simulink model "diagrama_LTI_desagragado"  (R2020b)
settings: Solver=VariableStepAuto  StartTime=0.0  StopTime=1.3  RelTol=1e-3
model workspace (MAT data in the model file):
  Cts = 0.818
  Jeq = 5.65099476805e-06
  Ld = 0.0066
  Lls = 0.0008
  Lq = 0.0058
  Pp = 3
  Rs = 1.02
  Rts_amb = 146.7
  beq = 1.5e-05
  lambda_m = 0.01546
  r = 314.3008
undefined symbols (not defined in the file or in its folder): sigbuilder_block
settings Model: Creator=Matias  LastModifiedBy=Matias

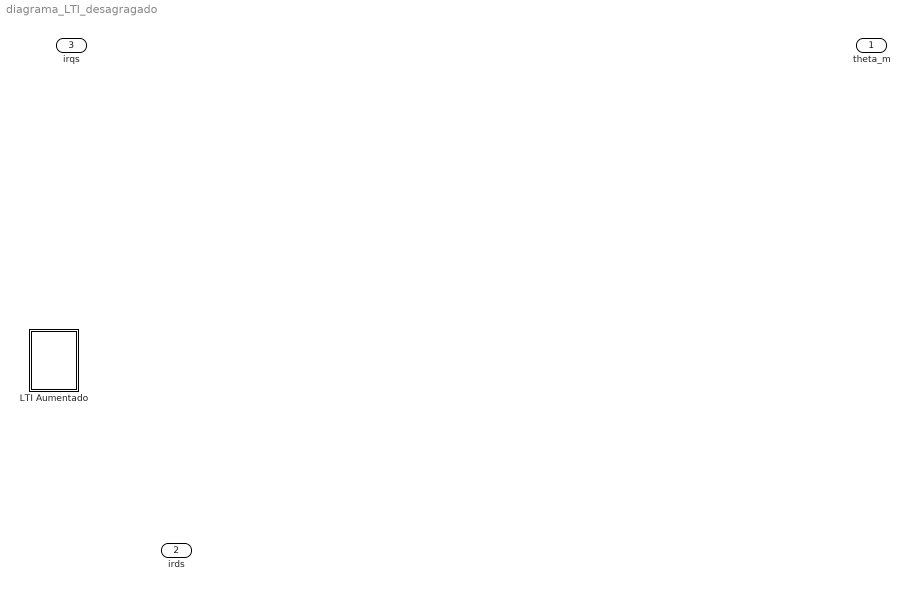
== system diagrama_LTI_desagragado ==
  LTI Aumentado : Subsystem
  theta_m : Outport
  irds : Outport  Port=2
  irqs : Outport  Port=3

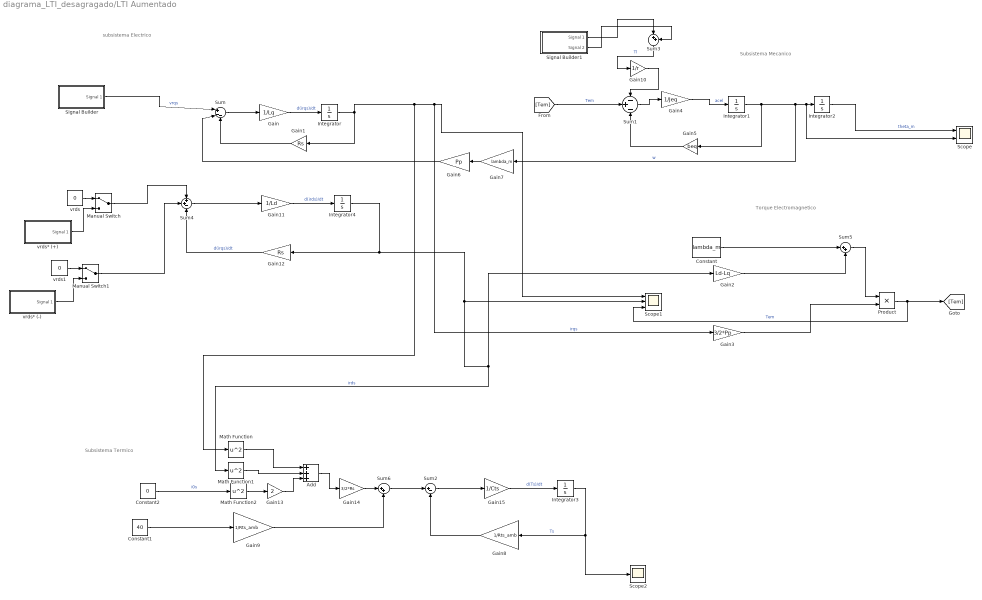
== system diagrama_LTI_desagragado/LTI Aumentado ==
  note: Subsistema Mecanico
  note: subsistema Electrico
  note: Subsistema Termico
  note: Torque Electromagnetico
  Add : Sum  Inputs=+++
  Constant : Constant  Value=lambda_m
  Constant1 : Constant  Value=40
  Constant2 : Constant  Value=0
  Gain : Gain  Gain=1/Lq
  Gain1 : Gain  Gain=Rs
  Gain10 : Gain  Gain=1/r
  Gain11 : Gain  Gain=1/Ld
  Gain12 : Gain  Gain=Rs
  Gain13 : Gain  Gain=2
  Gain14 : Gain  Gain=3/2*Rs
  Gain15 : Gain  Gain=1/Cts
  Gain2 : Gain  Gain=Ld-Lq
  Gain3 : Gain  Gain=3/2*Pp
  Gain4 : Gain  Gain=1/Jeq
  Gain5 : Gain  Gain=beq
  Gain6 : Gain  Gain=Pp
  Gain7 : Gain  Gain=lambda_m
  Gain8 : Gain  Gain=1/Rts_amb
  Gain9 : Gain  Gain=1/Rts_amb
  Integrator{,1..2,4} (4 alike) : Integrator
  Integrator3 : Integrator  InitialCondition=40
  Manual Switch : ManualSwitch
  Manual Switch1 : ManualSwitch
  Math Function : Math  Operator=square  SaturateOnIntegerOverflow=on
  Math Function1 : Math  Operator=square  SaturateOnIntegerOverflow=on
  Math Function2 : Math  Operator=square  SaturateOnIntegerOverflow=on
  Product : Product
  Scope : Scope  NumInputPorts=2
  Scope1 : Scope  NumInputPorts=3
  Scope2 : Scope
  Signal Builder : Subsystem  Tag=STV Subsys  LoadFcn=sigbuilder_block('load');  StartFcn=sigbuilder_block('start');  StopFcn=sigbuilder_block('stop');  ClipboardFcn=sigbuilder_block('clipboard');  mask(Sigbuilder block){tuvar=[0:10]}
      mask help: Simulink:masks:SigbuilderBlock_MD
      mask init:
      | if ~strcmp(get_param(bdroot(gcbh),'SimulationStatus'),'stopped') tuvar = sigbuilder_block('maskInit'); end
      settings: CopyFcn=sigbuilder_block('copy');  DeleteFcn=sigbuilder_block('delete');  ModelCloseFcn=sigbuilder_block('modelClose');  PreSaveFcn=sigbuilder_block('preSave');  PauseFcn=sigbuilder_block('pause');  ContinueFcn=sigbuilder_block('continue');  NameChangeFcn=sigbuilder_block('namechange');  OpenFcn=sigbuilder_block('open',[437.6 199.2 550.4 400 ]);  CloseFcn=sigbuilder_block('close');
      mask Display: plot(0, 0, 100, 100,[2, 2, 32, 32, 2], [68, 8, 8, 68, 68],[32, 2], [38, 38], [32, 19, 2],[53, 60, 44], [32, 17, 17, 2],[16, 16, 31, 31]);txt = getActiveGroup(gcbh);text(2, 100, txt,'verticalAlignment', 'top');
  Signal Builder1 : Subsystem  Tag=STV Subsys  LoadFcn=sigbuilder_block('load');  StartFcn=sigbuilder_block('start');  StopFcn=sigbuilder_block('stop');  ClipboardFcn=sigbuilder_block('clipboard');  mask(Sigbuilder block){tuvar=[0:10]}
      mask help: Simulink:masks:SigbuilderBlock_MD
      mask init:
      | if ~strcmp(get_param(bdroot(gcbh),'SimulationStatus'),'stopped') tuvar = sigbuilder_block('maskInit'); end
      settings: CopyFcn=sigbuilder_block('copy');  DeleteFcn=sigbuilder_block('delete');  ModelCloseFcn=sigbuilder_block('modelClose');  PreSaveFcn=sigbuilder_block('preSave');  PauseFcn=sigbuilder_block('pause');  ContinueFcn=sigbuilder_block('continue');  NameChangeFcn=sigbuilder_block('namechange');  OpenFcn=sigbuilder_block('open',[437.6 199.2 550.4 400 ]);  CloseFcn=sigbuilder_block('close');
      mask Display: plot(0, 0, 100, 100,[2, 2, 32, 32, 2], [68, 8, 8, 68, 68],[32, 2], [38, 38], [32, 19, 2],[53, 60, 44], [32, 17, 17, 2],[16, 16, 31, 31]);txt = getActiveGroup(gcbh);text(2, 100, txt,'verticalAlignment', 'top');
  Sum : Sum  Inputs=|+--
  Sum1 : Sum  Inputs=-+-
  Sum2 : Sum  Inputs=|+-
  Sum3 : Sum  Inputs=|++
  Sum4 : Sum  Inputs=++-
  Sum5 : Sum  Inputs=|++
  Sum6 : Sum  Inputs=|++
  vrds : Constant  Value=0
  vrds* (+) : Subsystem  Tag=STV Subsys  LoadFcn=sigbuilder_block('load');  StartFcn=sigbuilder_block('start');  StopFcn=sigbuilder_block('stop');  ClipboardFcn=sigbuilder_block('clipboard');  mask(Sigbuilder block){tuvar=[0:10]}
      mask help: Simulink:masks:SigbuilderBlock_MD
      mask init:
      | if ~strcmp(get_param(bdroot(gcbh),'SimulationStatus'),'stopped') tuvar = sigbuilder_block('maskInit'); end
      settings: CopyFcn=sigbuilder_block('copy');  DeleteFcn=sigbuilder_block('delete');  ModelCloseFcn=sigbuilder_block('modelClose');  PreSaveFcn=sigbuilder_block('preSave');  PauseFcn=sigbuilder_block('pause');  ContinueFcn=sigbuilder_block('continue');  NameChangeFcn=sigbuilder_block('namechange');  OpenFcn=sigbuilder_block('open',[437.6 199.2 550.4 400 ]);  CloseFcn=sigbuilder_block('close');
      mask Display: plot(0, 0, 100, 100,[2, 2, 32, 32, 2], [68, 8, 8, 68, 68],[32, 2], [38, 38], [32, 19, 2],[53, 60, 44], [32, 17, 17, 2],[16, 16, 31, 31]);txt = getActiveGroup(gcbh);text(2, 100, txt,'verticalAlignment', 'top');
  vrds* (-) : Subsystem  Tag=STV Subsys  LoadFcn=sigbuilder_block('load');  StartFcn=sigbuilder_block('start');  StopFcn=sigbuilder_block('stop');  ClipboardFcn=sigbuilder_block('clipboard');  mask(Sigbuilder block){tuvar=[0:10]}
      mask help: Simulink:masks:SigbuilderBlock_MD
      mask init:
      | if ~strcmp(get_param(bdroot(gcbh),'SimulationStatus'),'stopped') tuvar = sigbuilder_block('maskInit'); end
      settings: CopyFcn=sigbuilder_block('copy');  DeleteFcn=sigbuilder_block('delete');  ModelCloseFcn=sigbuilder_block('modelClose');  PreSaveFcn=sigbuilder_block('preSave');  PauseFcn=sigbuilder_block('pause');  ContinueFcn=sigbuilder_block('continue');  NameChangeFcn=sigbuilder_block('namechange');  OpenFcn=sigbuilder_block('open',[437.6 199.2 550.4 400 ]);  CloseFcn=sigbuilder_block('close');
      mask Display: plot(0, 0, 100, 100,[2, 2, 32, 32, 2], [68, 8, 8, 68, 68],[32, 2], [38, 38], [32, 19, 2],[53, 60, 44], [32, 17, 17, 2],[16, 16, 31, 31]);txt = getActiveGroup(gcbh);text(2, 100, txt,'verticalAlignment', 'top');
  vrds1 : Constant  Value=0
  wires:
  Gain7/1 -> Gain6/1
  Sum/1 -> Gain/1
  Integrator1/1 -> Gain7/1, Scope/2, Integrator2/1, Gain5/1  "w"
  Gain3/1 -> Product/2
  Integrator2/1 -> Scope/1  "theta_m"
  Gain15/1 -> Integrator3/1  "d(Ts)/dt"
  Integrator/1 -> Math Function/1, Gain3/1, Scope1/1, Gain1/1  "irqs"
  Gain4/1 -> Integrator1/1  "acel"
  Constant1/1 -> Gain9/1
  Gain5/1 -> Sum1/3
  Integrator4/1 -> Math Function1/1, Gain2/1, Scope1/2, Gain12/1  "irds"
  Sum4/1 -> Gain11/1
  Gain6/1 -> Sum/2
  Sum3/1 -> Gain10/1  "Tl"
  Gain11/1 -> Integrator4/1  "d(irds)/dt"
  Gain2/1 -> Sum5/2
  Constant/1 -> Sum5/1
  vrds* (+)/1(Signal 1) -> Manual Switch/2
  Sum2/1 -> Gain15/1
  vrds/1 -> Manual Switch/1
  Manual Switch/1 -> Sum4/1
  Gain14/1 -> Sum6/1
  Signal Builder1/1(Signal 1) -> Sum3/1
  Gain13/1 -> Add/3
  Product/1 -> Scope1/3, [Tem]  "Tem"
  vrds1/1 -> Manual Switch1/1
  Gain12/1 -> Sum4/3  "d(irqs)/dt"
  Gain10/1 -> Sum1/1
  Gain8/1 -> Sum2/2
  vrds* (-)/1(Signal 1) -> Manual Switch1/2
  Integrator3/1 -> Gain8/1, Scope2/1  "Ts"
  Signal Builder/1(Signal 1) -> Sum/1  "vrqs"
  Manual Switch1/1 -> Sum4/2
  Add/1 -> Gain14/1
  Signal Builder1/2(Signal 2) -> Sum3/2
  Math Function1/1 -> Add/2
  [Tem] -> Sum1/2  "Tem"
  Gain9/1 -> Sum6/2
  Sum6/1 -> Sum2/1
  Sum5/1 -> Product/1
  Sum1/1 -> Gain4/1
  Gain1/1 -> Sum/3
  Math Function/1 -> Add/1
  Math Function2/1 -> Gain13/1
  Gain/1 -> Integrator/1  "d(irqs)/dt"
  Constant2/1 -> Math Function2/1  "i0s"

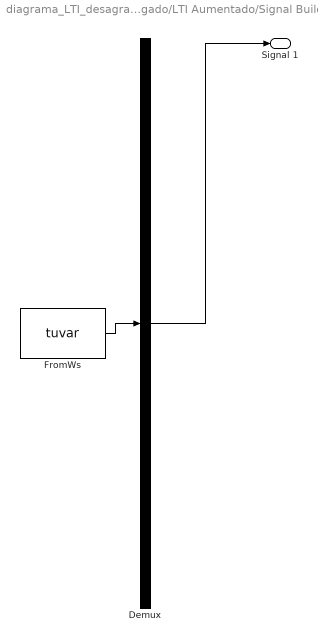
== system diagrama_LTI_desagragado/LTI Aumentado/Signal Builder ==
  Demux : Demux  Tag=STV Demux  Outputs=1
      settings: DisplayOption=none
  FromWs : FromWorkspace  Tag=STV FromWs  VariableName=tuvar
      SigBuilderData=|
      | common.afterFinalStr = 'Extrapolate'
      | common.sampleTime = 0
      | dataSet.timeRange = [0 10]
      | dataSet.name = 'Group 1'
      | sbobj.Groups.Name = 'Group 1'
      | sbobj.Groups.Signals.Name = 'Signal 1'
      | sbobj.Groups.Signals.XData = [0 0.1 0.1 0.7 0.7 10]
      | sbobj.Groups.Signals.YData = [0 0 19.596 19.596 0 0]
  Signal 1 : Outport  Tag=STV Outport
  wires:
  Demux/1 -> Signal 1/1
  FromWs/1 -> Demux/1

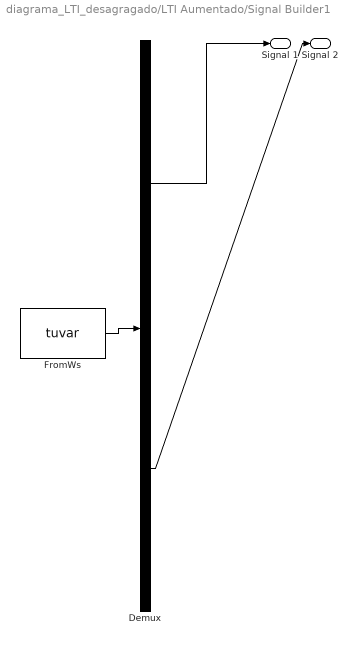
== system diagrama_LTI_desagragado/LTI Aumentado/Signal Builder1 ==
  Demux : Demux  Tag=STV Demux  Outputs=2
      settings: DisplayOption=none
  FromWs : FromWorkspace  Tag=STV FromWs  VariableName=tuvar
      SigBuilderData=|
      | common.afterFinalStr = 'Extrapolate'
      | common.sampleTime = 0
      | dataSet.timeRange = [0 10]
      | dataSet.name = 'Group 1'
      | sbobj.Groups.Name = 'Group 1'
      | sbobj.Groups.Signals(1).Name = 'Signal 1'
      | sbobj.Groups.Signals(1).XData = [0 0.3 0.3 0.5 0.5 10]
      | sbobj.Groups.Signals(1).YData = [0 0 6.28 6.28 0 0]
      | sbobj.Groups.Signals(2).Name = 'Signal 2'
      | sbobj.Groups.Signals(2).XData = [0 0.5 0.5 0.9 0.9 10]
      | sbobj.Groups.Signals(2).YData = [0 0 -6.28 -6.28 0 0]
  Signal 1 : Outport  Tag=STV Outport
  Signal 2 : Outport  Tag=STV Outport  Port=2
  wires:
  Demux/1 -> Signal 1/1
  FromWs/1 -> Demux/1
  Demux/2 -> Signal 2/1

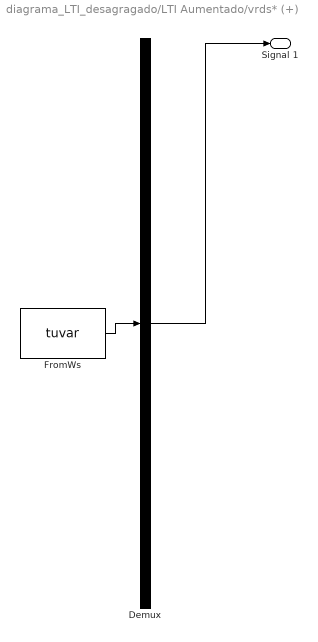
== system diagrama_LTI_desagragado/LTI Aumentado/vrds* (+) ==
  Demux : Demux  Tag=STV Demux  Outputs=1
      settings: DisplayOption=none
  FromWs : FromWorkspace  Tag=STV FromWs  VariableName=tuvar
      SigBuilderData=|
      | common.afterFinalStr = 'Extrapolate'
      | common.sampleTime = 0
      | dataSet.timeRange = [0 10]
      | dataSet.name = 'Group 1'
      | sbobj.Groups.Name = 'Group 1'
      | sbobj.Groups.Signals.Name = 'Signal 1'
      | sbobj.Groups.Signals.XData = [0 0.5 0.5 6 10]
      | sbobj.Groups.Signals.YData = [0 0 1.9596 1.9596 1.9596]
  Signal 1 : Outport  Tag=STV Outport
  wires:
  Demux/1 -> Signal 1/1
  FromWs/1 -> Demux/1

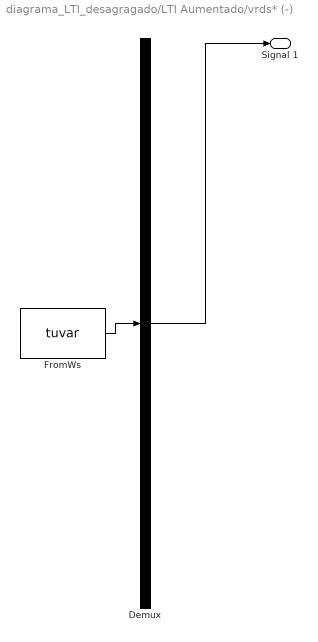
== system diagrama_LTI_desagragado/LTI Aumentado/vrds* (-) ==
  Demux : Demux  Tag=STV Demux  Outputs=1
      settings: DisplayOption=none
  FromWs : FromWorkspace  Tag=STV FromWs  VariableName=tuvar
      SigBuilderData=|
      | common.afterFinalStr = 'Extrapolate'
      | common.sampleTime = 0
      | dataSet.timeRange = [0 10]
      | dataSet.name = 'Group 1'
      | sbobj.Groups.Name = 'Group 1'
      | sbobj.Groups.Signals.Name = 'Signal 1'
      | sbobj.Groups.Signals.XData = [0 0.5 0.5 6 10]
      | sbobj.Groups.Signals.YData = [0 0 -1.9596 -1.9596 -1.9596]
  Signal 1 : Outport  Tag=STV Outport
  wires:
  Demux/1 -> Signal 1/1
  FromWs/1 -> Demux/1
